simulink model "Stabilization_Simulink_Offline_Pendulum_Control"  (R2019b)
settings: Solver=VariableStepAuto  StartTime=0.0  StopTime=30  RelTol=1e-3
values from neighbouring files (symbols this model uses):
  A = reshape([0.0,0.0,0.0,0.0,0.0,0.0,g.*m_p.*r.*t6.*t8,g.*l_p.*m_p.*t6.*t11,1.0,0.0,-t6.*t7.*t10.*t13,-l_p.*m_p.*r.*t6.*t7.*t13,0.0,1.0,-B_p.*l_p.*m_p.*r.*t6,-B_p.*t6.*t11],[4,4])    [SS_Matrices_Voltage_Unstable.m]
  B = [0.0;0.0;K_g.*eta_g.*eta_m.*k_t.*t6.*t7.*t10;K_g.*eta_g.*eta_m.*k_t.*l_p.*m_p.*r.*t6.*t7]    [SS_Matrices_Voltage_Unstable.m]
  C = eye(4)    [PolePlacement.m]    (also in SS_Matrices_Voltage_Unstable.m = reshape([1.0,0.0,0.0,1.0,0.0,0.0,0.0,0.0],[2,4]))
  D = zeros(4,1)    [PolePlacement.m]    (also in SS_Matrices_Voltage_Unstable.m = [0.0;0.0])
  voltage_max = 6    [PolePlacement.m]
undefined symbols (not defined in the file or in its folder): A_ob, B_ob, C_ob, D_ob, Kpp
libraries: simulink_extras x1
settings Model: Creator=utente  LastModifiedBy=Student

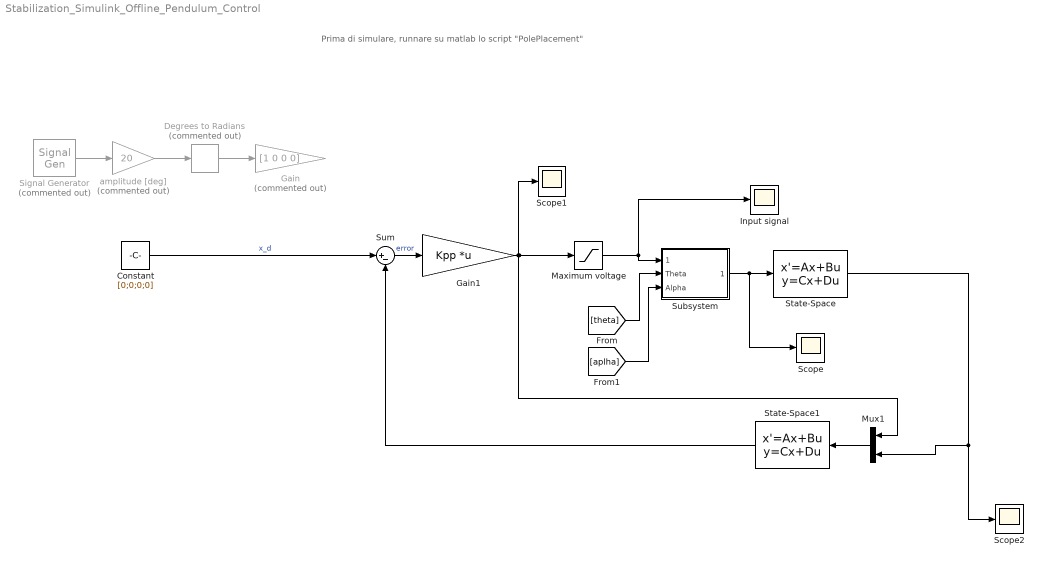
== system Stabilization_Simulink_Offline_Pendulum_Control ==
  note: Prima di simulare, runnare su matlab lo script "PolePlacement"
  Constant : Constant  Value=[0;0;0;0]
  Degrees to Radians : simulink_extras/Transformations/Degrees to Radians  Commented=on
  Gain : Gain  Commented=on  Gain=[1 0 0 0]
  Gain1 : Gain  Gain=Kpp  Multiplication=Matrix(K*u) (u vector)
  Input signal : Scope
  Maximum voltage : Saturate  UpperLimit=voltage_max  LowerLimit=-voltage_max
  Mux1 : Mux  Inputs=2
  Scope : Scope
  Scope1 : Scope
  Scope2 : Scope
  Signal Generator : SignalGenerator  Commented=on  Frequency=0.1
  State-Space : StateSpace  A=A  B=B  C=C  D=D  InitialCondition=[0 0.1 0 0]
  State-Space1 : StateSpace  A=A_ob  B=B_ob  C=C_ob  D=D_ob  InitialCondition=0
  Subsystem : Subsystem
  Sum : Sum  Inputs=|+-
  amplitude [deg] : Gain  Commented=on  Gain=20
  wires:
  Maximum voltage/1 -> Input signal/1, Subsystem/1(Control)
  Signal Generator/1 -> amplitude [deg]/1
  Sum/1 -> Gain1/1  "error"
  amplitude [deg]/1 -> Degrees to Radians/1
  Degrees to Radians/1 -> Gain/1
  [theta] -> Subsystem/2(Theta)
  [aplha] -> Subsystem/3(Alpha)
  Subsystem/1(control) -> State-Space/1, Scope/1
  Mux1/1 -> State-Space1/1
  State-Space/1 -> Scope2/1, Mux1/2
  Constant/1 -> Sum/1  "x_d"
  Gain1/1 -> Mux1/1, Scope1/1, Maximum voltage/1
  State-Space1/1 -> Sum/2

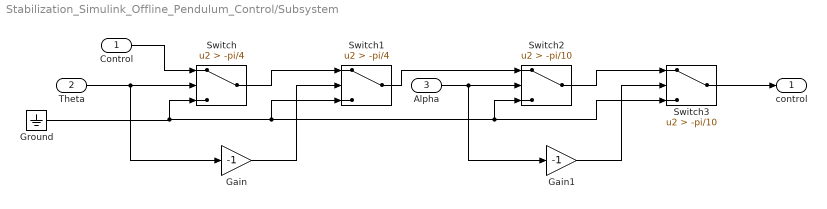
== system Stabilization_Simulink_Offline_Pendulum_Control/Subsystem ==
  Control : Inport
  Theta : Inport  Port=2
  Alpha : Inport  Port=3
  Gain : Gain  Gain=-1
  Gain1 : Gain  Gain=-1
  Ground : Ground
  Switch : Switch  Criteria=u2 > Threshold  Threshold=-pi/4
  Switch1 : Switch  Criteria=u2 > Threshold  Threshold=-pi/4
  Switch2 : Switch  Criteria=u2 > Threshold  Threshold=-pi/10
  Switch3 : Switch  Criteria=u2 > Threshold  Threshold=-pi/10
  control : Outport
  wires:
  Gain/1 -> Switch1/2
  Theta/1 -> Gain/1, Switch/2
  Control/1 -> Switch/1
  Switch/1 -> Switch1/1
  Gain1/1 -> Switch3/2
  Switch1/1 -> Switch2/1
  Ground/1 -> Switch3/3, Switch2/3, Switch1/3, Switch/3
  Switch2/1 -> Switch3/1
  Alpha/1 -> Switch2/2, Gain1/1
  Switch3/1 -> control/1
